simulink model "lab6_sim"  (R2024a)
settings: Solver=FixedStepAuto  StartTime=0.0  StopTime=25  FixedStep=0.01  RelTol=1e-3
settings Model: Creator=ventus  LastModifiedBy=ventus

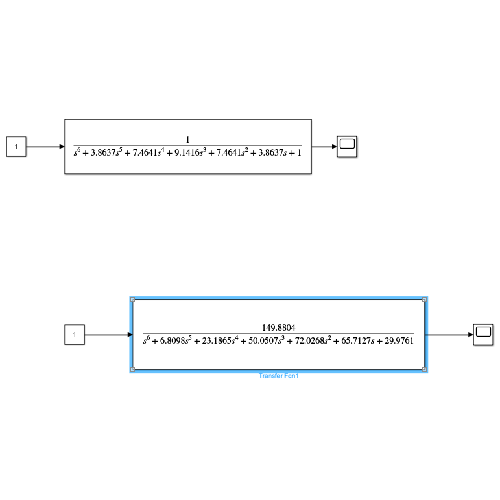
[thumbnail: Simulink's stored preview of the top-level diagram]
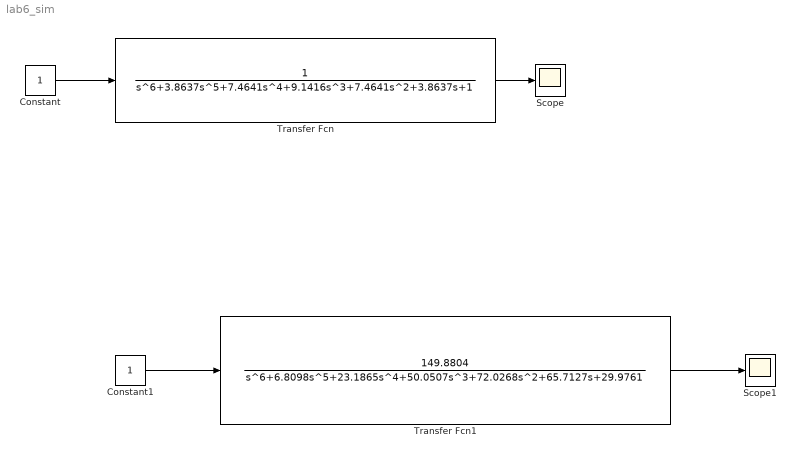
== system lab6_sim ==
  Constant : Constant
  Constant1 : Constant
  Scope : Scope
  Scope1 : Scope
  Transfer Fcn : TransferFcn  Denominator="[1 3.8637   7.4641  9.1416   7.4641   3.8637 1]"
  Transfer Fcn1 : TransferFcn  Numerator=[149.8804]  Denominator=[1 6.8098 23.1865 50.0507 72.0268 65.7127 29.9761]
  wires:
  Constant/1 -> Transfer Fcn/1
  Transfer Fcn/1 -> Scope/1
  Constant1/1 -> Transfer Fcn1/1
  Transfer Fcn1/1 -> Scope1/1
